simulink model "Kronecker_Ex1"  (R2025a)
settings: Solver=VariableStepAuto  StartTime=0.0  StopTime=10  RelTol=1e-3
undefined symbols (not defined in the file): Correlation_ValidMode, DUT, L, vsva1596, xcvc1702
libraries: aieDSP x1, vmcUtilities x1
settings Model: Creator=sdegala  LastModifiedBy=sdegala
settings ModelReferenceCC: EnableRefExpFcnMdlSchedulingChecks=on
settings RTWCC: GPUComputeCapability=3.5

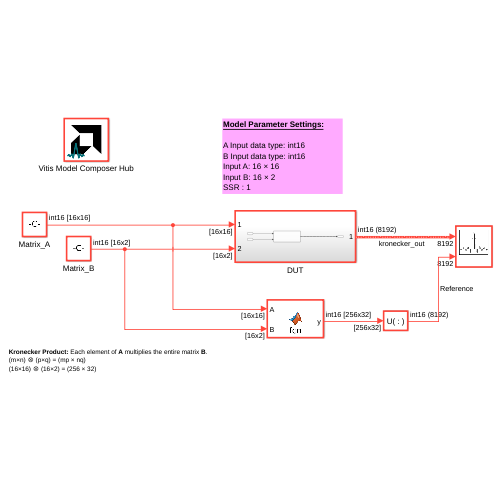
[thumbnail: Simulink's stored preview of the top-level diagram]
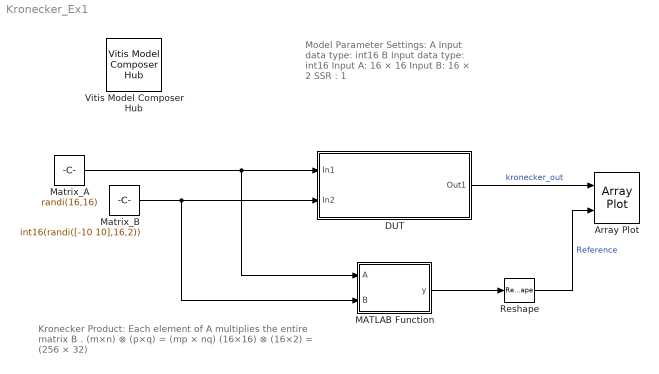
== system Kronecker_Ex1 ==
  note: Kronecker Product: Each element of A multiplies the entire matrix B .
      | (m×n) ⊗ (p×q) = (mp × nq)
      | (16×16) ⊗ (16×2) = (256 × 32)
  note: Model Parameter Settings:
      |
      | A Input data type: int16
      | B Input data type: int16
      | Input A: 16 × 16
      | Input B: 16 × 2
      | SSR : 1
  Array Plot : ArrayPlot  NumInputPorts=2  WindowPosition=[349.000000,449.000000,800.000000,500.000000,]  Visible=on  ScopeFrameLocation=window  YLimits=[-162 178]  ShowLegend=on
  DUT : Subsystem
  MATLAB Function : MATLAB Function  TreatAsAtomicUnit=on
  Matrix_A : Constant  Value=randi(16,16)  OutDataTypeStr=int16  SampleTime=1
  Matrix_B : Constant  Value=int16(randi([-10 10],16,2))  OutDataTypeStr=int16  SampleTime=1
  Reshape : Reshape
  Vitis Model Composer Hub : vmcUtilities/Vitis Model Composer Hub  Tag=genX  CodeGeneration=off  SubsystemName=DUT  BlockHierPath=Correlation_ValidMode/DUT  SubsystemType=AIENode  StartColumn=1  NumberOfColumns=1  TargetDirectory=./code  exportDesign=off  analyzeDesign=on  validateDesignOnHw=off  ExportType=AI Engines  IpVendor=xilinx.com  IpLibrary=hls  IpVersion=1.0  IpHWLanguage=Verilog  AieCompilerOptions={}  AieSimulatorOptions={}  CreateTestbench=on  TestbenchStackSize=10  RunRtlSim=off  RunCSim=off  RunAieSim=off  AieSimTimeout=50000  RunAieSimProfiling=off  LaunchVitisAnalyzer=off  PlotOutput=off  RunX86Sim=off  X86SimTimeout=10  GenHwImage=off  GenLibadfXo=off  GenHwValidationCode=off  PlatformType=Not Specified  HwSystemType=Baremetal  HwValidationTarget=hw  ProjDevice=xcvc1702-vsva1596-2LP-e-L  ProjDevicePart=xcvc1702-vsva1596-2LP-e-L  AIEType=AIE  SamplePeriod=-1  ClockFrequency=200  DataPathParallelism=1  xilinxfamily=versalaicore  part=xcvc1702  speed=-2LP-e-L  package=vsva1596  directory=./netlist  testbench=off  incr_netlist=off  synthesis_tool=Vivado  clock_wrapper=Clock Enables  dbl_ovrd=According to Block Masks  dcm_input_clock_period=10  sysclk_period=10  simulink_period=1  eval_field=0  IPInfoJsonString="{\"DUTSubsystemName\":\"DUT\",\"AIESubsystem\":{\"SubsystemName\":\"DUT\",\"TargetDirectory\":\"./code\",\"AIEArrayConfig\":\"Use entire AIE array\",\"StartColumn\":\"0\",\"NumberOfColumns\":\"1\"},\"SubsystemTag\":\"AIENode\"}"  LogFileName=/proj/xhdhdstaff5/sdegala/Head1/HEAD/2025_2_work/AIE_BLOCKS_2025_2/code/model_composer.log  NThreads=4  IPConfigFile=/tmp/vmctmp-11198269997411262707/Correlation_ValidMode_ipconfig.json
  wires:
  MATLAB Function/1(y) -> Reshape/1
  DUT/1(Out1) -> Array Plot/1  "kronecker_out"
  Matrix_A/1 -> MATLAB Function/1(A), DUT/1(In1)
  Matrix_B/1 -> MATLAB Function/2(B), DUT/2(In2)
  Reshape/1 -> Array Plot/2  "Reference"

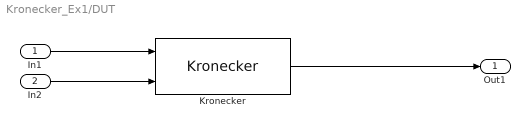
== system Kronecker_Ex1/DUT ==
  In1 : Inport
  In2 : Inport  Port=2
  Kronecker : aieDSP/Kronecker  AIE_VARIANT=1  TP_API=0  data_type_A=int16  data_type_B=int16  dim_a_rows=16  dim_a_cols=16  dim_b_rows=16  dim_b_cols=2  num_frames=1  shift_output=0  ssr=1  rnd_mode=Floor  sat_mode=None  blockJsonConstraints=[]  blockJsonConstraintsInternal=[]  spec=vmc_kronecker.json  SerializedMaskParamNames=[]  SerializedMaskParamValues=[]  SerializedMaskParamVisibilities=[]  block_type=Kronecker  SerializedMaskParamDataypes=uint|uint|typename|typename|uint|uint|uint|uint|uint|uint|uint|uint|uint  SerializedMaskParamEnumStrArr=0|0|0|0|0|0|0|0|0|0|0|Floor,Ceiling,Round to positive infinity,Round to negative infinity,Round symmetrical to infinity,Round symmetrical to zero,Round convergent to even,Round convergent to odd|None,Saturate,Symmetric  SerializedMaskParamEnumValArr=0|0|0|0|0|0|0|0|0|0|0|0,1,2,3,4,5,6,7|0,1,3  SerializedMaskParamVectorArr=0|0|0|0|0|0|0|0|0|0|0|0|0  SerializedMaskParamKeys=AIE_VARIANT|TP_API|TT_DATA_A|TT_DATA_B|TP_DIM_A_ROWS|TP_DIM_A_COLS|TP_DIM_B_ROWS|TP_DIM_B_COLS|TP_NUM_FRAMES|TP_SHIFT|TP_SSR|TP_RND|TP_SAT
  Out1 : Outport
  wires:
  In2/1 -> Kronecker/2
  In1/1 -> Kronecker/1
  Kronecker/1 -> Out1/1

== matlab function Kronecker_Ex1/MATLAB Function ==
  data: A input; y output; B input
 function y = fcn(A,B)
  y = kron(A,B);
